simulink model "Noa_Nofusion_backup"  (R2020b)
settings: Solver=FixedStepDiscrete  StartTime=0.0  StopTime=Inf  FixedStep=0.02  RelTol=1e-3
PostLoadFcn:
  | if any(exist('dsrtsu_mdlpostloadfcn', 'file') ~= 0), dsrtsu_mdlpostloadfcn('Execute', bdroot); end
InitFcn:
  | , if any(exist('rtifpga_mdlclblib', 'file') ~= 0), rtifpga_mdlclblib('Init', bdroot); end,
  | , if any(exist('dsmpb_private', 'file') ~= 0), dsmpb_private('dsmpb_mdlclblib', 'Init', bdroot); end,
undefined symbols (not defined in the file): ACC_TimeGap_DecSetSwt, ACC_TimeGap_IncSetSwt, AccelPedalPosn, AccelPedalPosnVldty, AccelPedlPosnDiagc, AccPedalOverride, ACU_ShiftInProgress, ADAS_Posn_CurLane, AESSwtReq, ALC_SwtReq, BrkPedalSts, CC_ACC_CANCEL_OFFSwt, CC_ACC_CRUISE_OFFSwt, CC_ACC_DecSetSpd_SetSwt, CC_ACC_IncSetSpd_ResuSwt, CC_ACCSwtErr, CharSpd_ms, CSA_NODE, CURRENT_GEAR, CurrentGearValid, DiscIntNeverNeededParam, DrvDoorSts, DrvSBR, DrvTrqReqOvld, ECMACCInterface, ECMRespACC, ELKSwtReq, EngLimpHomeSts, EngSpd, EngState, EngState_PHEV, EngTrqMaxActSpd, EngTrqMinAct, EPS_DrvInpTrqVal_HighReslolution, EPS_FailSts, EPS_LKATorqOvrlDlvd, EPS_LKATorqOvrlDlvdVld, EPS_LKATrqOvlDlvdSts, EPS_SteerMod, EPS_TrqSnsrSts, EQ4_APPINFO, EQ4_LA_ELEM, EQ4_LA_HDR, EQ4_LAP_ELEM, EQ4_LAP_HDR, EQ4_LH_ELEM, EQ4_LH_HDR, EQ4_LRE_ELEM, EQ4_LRE_HDR, ESS_PedSwtReq, ESS_VehSwtReq, FFogLmpSts_F_Pbox, FLWheelDriveDirection, FLWheelSpd, FrntWiprSwtSts, FrntWshrSwtSts, FRWheelDriveDirection, FRWheelSpd, HazardLmpSwtSts, HCU_AccelPedalPosn_Diag ... (+152)
libraries: simulink x117, dsmpblib x30
(part 10 of 11)

== matlab function Noa_Nofusion_backup/Subsystem2/ACCOSM/HWA_Task100ms1/Trajectory/Trajectory/CalcEgoVehMove ==
  data: dDeltaX output single size=1; tCycle input size=1; Kap input size=1; Vego input size=1; alpSideSlipAngle input size=1; dDeltaY output single size=1; CosOfPsi output single size=1; SinOfPsi output single size=1; WheelTrack input; SlipDislim output; Vch input
function [dDeltaX,dDeltaY,CosOfPsi,SinOfPsi,SlipDislim] = EgoVehicleMovement(tCycle,Kap,Vego,alpSideSlipAngle,WheelTrack,Vch)
%#codegen
if Kap==0
    dDeltaX = Vego*tCycle;
    dDeltaY = single(0);
    CosOfPsi = single(1);
    SinOfPsi = single(0);
    SlipDislim = Vch*1000;
else
    SlipDislim = max(WheelTrack*1000,min(tCycle*Vego,Kap*15));
    t_Psi = Kap*Vego*tCycle;
    SinOfPsi = sin(t_Psi);
    CosOfPsi = cos(t_Psi);
    t_dDeltaXTemp = SinOfPsi/Kap;
    t_dDeltaYTemp = 2*(sin(t_Psi/2)*sin(t_Psi/2))/Kap;
    dDeltaX = min(cos(alpSideSlipAngle)*t_dDeltaXTemp - sin(alpSideSlipAngle)*t_dDeltaYTemp,SlipDislim);
    dDeltaY = sin(alpSideSlipAngle)*t_dDeltaXTemp + cos(alpSideSlipAngle)*t_dDeltaYTemp;
end

== matlab function Noa_Nofusion_backup/Subsystem2/ACCOSM/HWA_Task100ms1/Trajectory/Trajectory/Priority ==
  data: ObjNumber input; ObjValid input; ObjPrio output single; ObjClass input; ObjDx input; ObjMatrix output single
function [ObjPrio,ObjMatrix] = fcn(ObjNumber,ObjValid,ObjClass,ObjDx)
%#codegen
ObjPrio = single(zeros(15,1));

for i=1:ObjNumber
    if ObjValid(i)
        if ObjDx(i)<0
            ObjPrio(i)=single(0);
        else
            if (ObjClass(i)==2)||(ObjClass(i)==3)||(ObjClass(i)==5)
                t_ObjPrio=single(2*255);
            else
                t_ObjPrio=single(255);
            end
            ObjPrio(i) = t_ObjPrio - ObjDx(i);
        end
    else
        ObjPrio(i)=single(0);
    end
end

ObjMatrix=ObjPrio;

t_h=1;
while 1
    t_h = t_h*3+1;
    if t_h>=ObjNumber
        break;
    end
end

%   t_h = 121;
while 1
    t_h = fix(t_h/3);
    for i=(t_h+1):ObjNumber
        j=i;
        t_zw=ObjMatrix(i);
        while (j>t_h)&&(t_zw<ObjMatrix(j-t_h))
            ObjMatrix(j)=ObjMatrix(j-t_h);
            j=j-t_h;
        end
        ObjMatrix(j)=t_zw;
    end
    if t_h==1
        break;
    end
end

== matlab function Noa_Nofusion_backup/Subsystem2/ACCOSM/HWA_Task100ms1/Trajectory/Trajectory/ReleaseLowPriorityObjects ==
  data: TrajUsed output; ObjNumber input; TrajNumber input; ObjPrio input; ObjMatrix input; ObjValid input; TrajCurrentIndex input; TrajUsedK1 input; TrajHistBufferBTrajEndK1 input; ObjTrajNumberK1 input; TrajHistBufferBTrajEnd output; ObjTrajNumber output
function [TrajUsed,TrajHistBufferBTrajEnd,ObjTrajNumber] =...
    fcn(ObjNumber,TrajNumber,ObjPrio,ObjMatrix,ObjValid,TrajCurrentIndex,...
    TrajUsedK1,TrajHistBufferBTrajEndK1,ObjTrajNumberK1)
%#codegen
TrajHistBufferBTrajEnd = TrajHistBufferBTrajEndK1;
TrajUsed = TrajUsedK1;
ObjTrajNumber = ObjTrajNumberK1;
ObjPrioLimit = ObjMatrix(ObjNumber-TrajNumber);

for i=1:ObjNumber
    if ObjValid(i)
        if (ObjPrio(i)==0)||(ObjPrio(i)<=ObjPrioLimit)
            j = ObjTrajNumber(i);
            if j<(TrajNumber+1)
                t = TrajCurrentIndex(j);
                TrajHistBufferBTrajEnd(j,t)=1;
                TrajUsed(j)=0;
                ObjTrajNumber(i)=255;
            end
        end
    end
end

== matlab function Noa_Nofusion_backup/Subsystem2/ACCOSM/HWA_Task100ms1/Trajectory/Trajectory/StoreEgoTrajectory ==
  data: Pa output single; Pb output single; Pc output single; Pd output single; BufNumber input; tCycle input; EgoTrajHistCurrentIndex output uint8; EgoDDeltaX input; EgoDDeltaY input; EgoCosOfPsi input; EgoSinOfPsi input; EgoTrajHistDxv output; EgoTrajHistDyv output; EgoTrajHistTTimeStamp output; EgoTrajHistCurrentIndexK1 input; EgoTrajHistDxvK1 input single; EgoTrajHistDyvK1 input single; EgoTrajHistTTimeStampK1 input single
function [Pa,Pb,Pc,Pd,EgoTrajHistCurrentIndex,EgoTrajHistDxv,EgoTrajHistDyv,EgoTrajHistTTimeStamp]...
    = fcn(BufNumber,tCycle,EgoDDeltaX,EgoDDeltaY,EgoCosOfPsi,EgoSinOfPsi,...
    EgoTrajHistCurrentIndexK1,EgoTrajHistDxvK1,EgoTrajHistDyvK1,EgoTrajHistTTimeStampK1)
%#codegen
EgoTrajHistCurrentIndex = EgoTrajHistCurrentIndexK1;
EgoTrajHistDxv = EgoTrajHistDxvK1;
EgoTrajHistDyv = EgoTrajHistDyvK1;
EgoTrajHistTTimeStamp = EgoTrajHistTTimeStampK1;
% alpWheelAngleOffset = alpWheelAngleOffsetK1;

t_IdxActualElement = EgoTrajHistCurrentIndex;
if t_IdxActualElement==BufNumber
    t_IdxNextElement=uint8(1);
else
    t_IdxNextElement=t_IdxActualElement+1;
end

Temp1 = EgoTrajHistDxv(t_IdxActualElement) - EgoDDeltaX;
Temp2 = EgoTrajHistDyv(t_IdxActualElement) - EgoDDeltaY;
dDeltaS = Temp1*Temp1 + Temp2*Temp2;
t_AddPosition = ((EgoTrajHistTTimeStamp(t_IdxActualElement)+tCycle)>0.3);
t_AddPosition = t_AddPosition&(dDeltaS>4);
t_AddPosition = t_AddPosition|(dDeltaS>100);
for iBuf=1:BufNumber
    if (t_AddPosition==1)&&(iBuf==t_IdxNextElement)
        EgoTrajHistDxv(iBuf)=single(0);
        EgoTrajHistDyv(iBuf)=single(0);
        EgoTrajHistTTimeStamp(iBuf)=single(0);
        EgoTrajHistCurrentIndex = t_IdxNextElement;
    else
        dX = EgoTrajHistDxv(iBuf)-EgoDDeltaX;
        dY = EgoTrajHistDyv(iBuf)-EgoDDeltaY;
        if (EgoTrajHistDxv(iBuf)>-255)&&(dX>-255)&&(dX<255)&&(dY>-255)&&(dY<255)
            Temp1 = dX*EgoCosOfPsi + dY*EgoSinOfPsi;
            Temp2 = -dX*EgoSinOfPsi + dY*EgoCosOfPsi;
            if (Temp1>-255)&&(Temp1<255)&&(Temp2>-255)&&(Temp2<255)
                EgoTrajHistDxv(iBuf)=Temp1;
                EgoTrajHistDyv(iBuf)=Temp2;
                tDt = EgoTrajHistTTimeStamp(iBuf)+tCycle;
                if tDt>32
                    tDt=single(32);
                end
                EgoTrajHistTTimeStamp(iBuf) = tDt;
            else
                EgoTrajHistDxv(iBuf)=single(-255);
                EgoTrajHistDyv(iBuf)=single(-255);
                EgoTrajHistTTimeStamp(iBuf) = single(32);
            end
        else
            EgoTrajHistDxv(iBuf)=single(-255);
            EgoTrajHistDyv(iBuf)=single(-255);
            EgoTrajHistTTimeStamp(iBuf) = single(32);
        end
    end
end

t_Index = EgoTrajHistCurrentIndex;
t_Index1 = BufNumber + uint8(23);
t_Index2 = BufNumber + uint8(21);
t_Index3 = BufNumber + uint8(19);

if t_Index1>24
    t_Index1 = t_Index1 - uint8(24);
end
if t_Index2>24
    t_Index2 = t_Index2 - uint8(24);
end
if t_Index3>24
    t_Index3 = t_Index3 - uint8(24);
end

XiMa = [EgoTrajHistDxv(t_Index);EgoTrajHistDxv(t_Index1);EgoTrajHistDxv(t_Index2);EgoTrajHistDxv(t_Index3)];
YiMa = [EgoTrajHistDyv(t_Index);EgoTrajHistDyv(t_Index1);EgoTrajHistDyv(t_Index2);EgoTrajHistDyv(t_Index3)];

[Pa,Pb,Pc,Pd] = pl(XiMa,YiMa);

% if (abs(EgoTrajHistDyv(t_Index1))<0.1)&&(abs(EgoTrajHistDyv(t_Index2))<0.1)&&(abs(EgoTrajHistDyv(t_Index3))<0.1)
%     kapRef = 3*Pa*EgoTrajHistDxv(t_Index2) + 2*Pb;
%     AckConst = min((1+VxvRef*VxvRef/(26*26))*2.68/max(VxvRef,1),32767);
%     alpWheelAngleRef = VxvRef*kapRef*AckConst;
%     Raw = alpWheelAngleMean - alpWheelAngleRef;
%     if VxvRef>7.3
%         alpWheelAngleOffset = (Raw - alpWheelAngleOffset)/10000 + alpWheelAngleOffset;
%     end
% else
%     alpWheelAngleRef = single(255);
% end

== matlab function Noa_Nofusion_backup/Subsystem2/ACCOSM/HWA_Task100ms1/VycCalc ==
  data: ObjVyc output single size=15; dxC0 input; aP0 input; bP0 input; aP1 input; bP1 input; ObjValid input boolean size=15; ObjDx input single size=15; ObjVxG input single size=15; ObjVyG input single size=15; ObjYawAngle output
function [ObjVyc,ObjYawAngle] = VycCalc(dxC0,aP0,bP0,aP1,bP1,ObjValid,ObjDx,ObjVxG,ObjVyG)

ObjVyc = single(zeros(15,1));
ObjYawAngle = single(zeros(15,1));

for i=1:15
    if ObjValid(i)
       t_dxv = ObjDx(i);
       t_VxG = ObjVxG(i);
       t_VyG = ObjVyG(i);
       
       if abs(t_VxG)<0.1
          if t_VyG>0.5
              ObjYawAngle(i) = single(1.57);
          end
          if t_VyG<-0.5
              ObjYawAngle(i) = single(-1.57);
          end
       else
           if t_VxG>0
               ObjYawAngle(i) = atan(t_VyG/t_VxG);
           else
               if t_VyG>0
                  ObjYawAngle(i) = single(3.1416) + atan(t_VyG/t_VxG);
               else
                  ObjYawAngle(i) = -single(3.1416) + atan(t_VyG/t_VxG);
               end
           end
       end
       
       t_bParabolaYNLane = single(1);
       if t_dxv<dxC0
          temp1 =  2*aP0*t_dxv + bP0;
          t_bParabolaXNLane = -temp1;
       else
          temp1 =  2*aP1*t_dxv + bP1;
          t_bParabolaXNLane = -temp1;
       end
       t_bParabolaMag = mag(t_bParabolaXNLane,t_bParabolaYNLane);
       t_bParabolaXNLane = t_bParabolaXNLane/t_bParabolaMag;
       t_bParabolaYNLane = t_bParabolaYNLane/t_bParabolaMag;
       temp1 = t_VxG*t_bParabolaXNLane;
       temp2 = t_VyG*t_bParabolaYNLane;
       
       ObjVyc(i) = temp1 + temp2;
    else
       ObjVyc(i) = single(0);
    end
end
end

function out = mag(x,y)
M = max(abs(x),abs(y));
N = min(abs(x),abs(y));
out = M + 0.322*N;
end

== matlab function Noa_Nofusion_backup/Subsystem2/ACCOSM/HWA_Task100ms1/dyLaneWidthSteerAdapt ==
  data: kap input; dyLaneAdaptLeft output; dyAdapt input; dyLaneAdaptRight output
function [dyLaneAdaptLeft,dyLaneAdaptRight] = fcn(kap,dyAdapt)

dyLaneAdaptLeft = single(0);
dyLaneAdaptRight = single(0);
if kap>0
    dyLaneAdaptRight = dyAdapt;
end
if kap<0
    dyLaneAdaptLeft = dyAdapt;
end

== matlab function Noa_Nofusion_backup/Subsystem2/ACCOSM/HWA_Task100ms1/wCutInVy ==
  data: DycASI output single; ObjValid input boolean size=15; ObjDycCutIn input single size=15; ObjWidth input single size=15; ObjVyc input single size=15; ObjDx input single size=15; ObjDy input single size=15; ObjCnt input uint8 size=15; ObjDycFilt input single size=15; ObjwCutInVyK1 input single size=15; ObjtPrediction4CutIn output single size=15; ObjDycCutInPredict output single size=15; ObjCutIn_b output boolean size=15; ObjwCutInVy output single size=15
function [DycASI,ObjtPrediction4CutIn,ObjDycCutInPredict,ObjCutIn_b,ObjwCutInVy] = ...
    CalcWCutInVy(ObjValid,ObjDycCutIn,ObjWidth,ObjVyc,ObjDx,ObjDy,ObjCnt,...
    ObjDycFilt,ObjwCutInVyK1)
 
ObjwCutInVy = single(zeros(15,1));
ObjtPrediction4CutIn = single(zeros(15,1));
ObjDycCutInPredict = single(zeros(15,1));
DycASI = single(zeros(15,1));
ObjCutIn_b = false(15,1);
 
for i=1:15
    if ObjValid(i)
        dWidth = ObjWidth(i);
        dycASI = ObjDycCutIn(i);
        vyc = ObjVyc(i);
        dx = ObjDx(i);
        dy = ObjDy(i);
        dycFilt = ObjDycFilt(i);
        wCutInVyK1 = ObjwCutInVyK1(i);
  
        temp1 = dycFilt - dycASI;
        if ((dycASI>0)&&(temp1>0.2))||((dycASI<0)&&(temp1<-0.2))
            tauVy = single(1.6);
        else
            tauVy = single(0);
        end
        tauVy = interpolate(single(40),tauVy,single(70),single(0),dx);
        ObjtPrediction4CutIn(i) = tauVy;
        temp1 = vyc*tauVy;
        temp2 = dycASI + temp1;
        
        if (dycASI>0)&&(temp2<0)
            temp2 = single(0);
        else
            if (dycASI<0)&&(temp2>0)
                temp2 = single(0);
            else
                if dycASI==0
                    temp2 = single(0);
                end
            end
        end
        ObjDycCutInPredict(i) = temp2;
        if dycASI>0
            temp1 = temp2 - 0.5*dWidth;
            t_dycASI = max(temp1,single(0));
        else
            temp1 = temp2 + 0.5*dWidth;
            t_dycASI = min(temp1,single(0));
        end
        temp1 = abs(t_dycASI);
        t_wCutInVy = interpolate(single(0),single(1),single(0.7),single(0),temp1);
        if tauVy==0
            t_wCutInVy = single(0);
        end
        
        if dx>0
            fak = abs(dy)/dx; 
        else
            fak = single(0);
        end
        if (ObjCnt(i)<2)||(abs(dy)>=2.4)||(fak>0.25)
           t_wCutInVy = single(0);
        end
       
        temp1 = t_wCutInVy - wCutInVyK1;
        temp1_ub = abs(temp1);
        temp2 = 0.2*temp1_ub;
        if temp1>0
            t_wCutInVy = wCutInVyK1 + temp2;
        else
            t_wCutInVy = wCutInVyK1 - temp2;
        end
        ObjwCutInVy(i) = t_wCutInVy;
        DycASI(i) = t_dycASI;
        if t_wCutInVy>0.7
            ObjCutIn_b(i) = true;
        end
    end
end
end
 
% function out = interpolate(x1,z1,x2,z2,Raw)
% if Raw<=x1
%     out = z1;
% else
%     if Raw>=x2
%         out = z2;
%     else
%         out = z1 + (Raw-x1)*(z2-z1)/(x2-x1);
%     end
% end
% end

== matlab function Noa_Nofusion_backup/Subsystem2/ACCOSM/HWA_Task100ms1/wCutOutVy ==
  data: vRef input single size=1; kap input single size=1; tDirIndLeft input single size=1; tDirIndRight input single size=1; ObjValid input boolean size=15; ObjDycCutIn input single size=15; ObjWidth input single size=15; ObjtPrediction4CutOut output single size=15; ObjDycCutOutPredict output single size=15; ObjwCutOutTurnOff output single size=15; ObjVyc input single size=15; ObjDx input single size=15; ObjDy input single size=15; ObjVx input single size=15; ObjVy input single size=15; ObjDyc input single size=15; ObjDrive_b input boolean size=15; ObjCnt input uint8 size=15; ObjDycFilt input single size=15; ObjwCutoutVyK1 input single size=15; ObjwCutoutVy output single size=15
function [ObjtPrediction4CutOut,ObjDycCutOutPredict,ObjwCutOutTurnOff,ObjwCutoutVy] = ...
    CalcWCutOutVy(vRef,kap,tDirIndLeft,tDirIndRight,ObjValid,ObjDycCutIn,ObjWidth,...
    ObjVyc,ObjDx,ObjDy,ObjVx,ObjVy,ObjDyc,ObjDrive_b,ObjCnt,...
    ObjDycFilt,ObjwCutoutVyK1)
 
ObjwCutoutVy = single(zeros(15,1));
ObjtPrediction4CutOut = single(zeros(15,1));
ObjDycCutOutPredict = single(zeros(15,1));
ObjwCutOutTurnOff = single(zeros(15,1));
 
for i=1:15
    if ObjValid(i)
        dWidth = ObjWidth(i);
        dycASI = ObjDycCutIn(i);
        vyc = ObjVyc(i);
        dx = ObjDx(i);
        dy = ObjDy(i);
        vx = ObjVx(i);
        vy = ObjVy(i);
        dyc = ObjDyc(i);
        dycFilt = ObjDycFilt(i);
        wCutoutVyK1 = ObjwCutoutVyK1(i);
        Move_b = ObjDrive_b(i);
        Cnt = ObjCnt(i);
        t_vxTO = vRef + vx;
        t_vxvThreshold = 0.5 - vRef;
        
        temp1 = dycASI - dycFilt;
        if ((dycASI>0)&&(temp1>0.2))||((dycASI<0)&&(temp1<-0.2))
            tauVy = single(1);
        else
            tauVy = single(0);
        end
        tauVy = interpolate(single(40),tauVy,single(70),single(0),dx);
        ObjtPrediction4CutOut(i) = tauVy;
        temp1 = vyc*tauVy;
        temp2 = dycASI + temp1;
        
        if (dycASI>0)&&(temp2<0)
            temp2 = single(0);
        else
            if (dycASI<0)&&(temp2>0)
                temp2 = single(0);
            else
                if dycASI==0
                    temp2 = single(0);
                end
            end
        end
        ObjDycCutOutPredict(i) = temp2;
        if dycASI>0
            temp1 = temp2 + 0.5*dWidth;
            t_dycASI = max(temp1,single(0));
        else
            temp1 = temp2 - 0.5*dWidth;
            t_dycASI = min(temp1,single(0));
        end
        temp1 = abs(t_dycASI);
        t_wCutoutVy = interpolate(single(0),single(0),single(0.7),single(1),temp1);
        if tauVy==0
            t_wCutoutVy = single(0);
        end
        
        temp1 = t_wCutoutVy - wCutoutVyK1;
        temp1_ub = abs(temp1);
        temp2 = 0.2*temp1_ub;
        if temp1>0
            t_wCutoutVy = wCutoutVyK1 + temp2;
        else
            t_wCutoutVy = wCutoutVyK1 - temp2;
        end
        ObjwCutoutVy(i) = t_wCutoutVy;
        if (dx<30)&&(Move_b==true)&&(vRef>0.5)&&(t_vxTO<6)&&(vx>t_vxvThreshold)&&(abs(dyc)>0.5)&&...
        (abs(dy)>0.5)&&(abs(dy)<4)&&(abs(vy)>0.5)&&...
        (((dyc<0)&&(vyc<0)&&(tDirIndRight==0))||((dyc>0)&&(vyc>0)&&(tDirIndLeft==0)))&&...
        (kap>-0.005)&&(kap<0.005)&&...
        (Cnt==7) 
             ObjwCutOutTurnOff(i) = t_wCutoutVy;
        end
    end
end
end

== matlab function Noa_Nofusion_backup/CR_RSDS_Input/CL ==
  data: ID input uint8 size=11; Dx input single size=11; Dy input single size=11; Vx input single size=11; Vy input single size=11; Ax input single size=11; Age input uint8 size=11; MoveSts input uint8 size=11; FusType input uint8 size=11; ObjIDK1 input uint8 size=11; ObjDx output single size=11; ObjDy output single size=11; ObjVx output single size=11; ObjVy output single size=11; ObjAx output single size=11; ObjAge output uint8 size=11; ObjMoveSts output uint8 size=11; ObjFusType output uint8 size=11; ObjID output uint8 size=11
function [ObjDx,ObjDy,ObjVx,ObjVy,ObjAx,ObjAge,ObjMoveSts,ObjFusType,ObjID] =...
    DataT(ID,Dx,Dy,Vx,Vy,Ax,Age,MoveSts,FusType,ObjIDK1)

ObjID = uint8(zeros(11,1));
ObjDx = single(zeros(11,1));
ObjDy = single(zeros(11,1));
ObjVx = single(zeros(11,1));
ObjVy = single(zeros(11,1));
ObjAx = single(zeros(11,1));
ObjAge = uint8(zeros(11,1));
ObjMoveSts = uint8(zeros(11,1));
ObjFusType = uint8(zeros(11,1));

T = uint8(zeros(11,1));
P = uint8(zeros(11,1));
Index01 = uint8(zeros(11,1));
Index02 = uint8(zeros(11,1));
M = uint8(0);
N = uint8(0);
w = uint8(0);

for i=uint8(1):uint8(11)
    for j=uint8(1):uint8(11)
        if ID(i)==ObjIDK1(j) && ID(i)>uint8(0)
            T(j) = i;
            P(i) = j;
        end
    end
end

for j=uint8(1):uint8(11)
    if T(j)==uint8(0)
        if ObjIDK1(j)==uint8(0)
            N = N + uint8(1);
            Index01(N) = j;
        else
            M = M + uint8(1);
            Index02(M) = j;
        end
    end
end

for i=uint8(1):uint8(11)
    if P(i)==uint8(0) && ID(i)>uint8(0)
        w = w + uint8(1);
        if w<=N
            P(i) = Index01(w);
        else
            P(i) = Index02(w - N);
        end
    end
    if P(i)>uint8(0)
       ObjID(P(i)) = ID(i);
       ObjDx(P(i)) = Dx(i);
       ObjDy(P(i)) = Dy(i);
       ObjVx(P(i)) = Vx(i);
       ObjVy(P(i)) = Vy(i);
       ObjAx(P(i)) = Ax(i);
       ObjAge(P(i)) = Age(i);
       ObjMoveSts(P(i)) = MoveSts(i);
       ObjFusType(P(i)) = FusType(i);
    end
end
end

== matlab function Noa_Nofusion_backup/CR_RSDS_Input/CR_L_Bus/CL ==
  data: RadarID input uint8 size=1; ID input uint8 size=6; Dx input single size=6; Dy input single size=6; Vx input single size=6; Vy input single size=6; Ax input single size=6; ObjIDK1 input uint8 size=6; P output uint8 size=6; ObjDx output single size=6; ObjDy output single size=6; ObjVx output single size=6; ObjVy output single size=6; ObjAx output single size=6; ObjMoveSts output uint8 size=6; ObjFusType output uint8 size=6; ObjID output uint8 size=6; ObjAgeK1 input uint8 size=6; ObjAge output uint8 size=6
function [P,ObjDx,ObjDy,ObjVx,ObjVy,ObjAx,ObjMoveSts,ObjFusType,ObjID,ObjAge] =...
    DataT(RadarID,ID,Dx,Dy,Vx,Vy,Ax,ObjIDK1,ObjAgeK1)

if RadarID==uint8(1)
    FusFac = 4;
elseif RadarID==uint8(2)
    FusFac = 8;
elseif RadarID==uint8(3)
    FusFac = 16;
else
    FusFac = 32;
end

ObjID = uint8(zeros(6,1));
ObjDx = single(zeros(6,1));
ObjDy = single(zeros(6,1));
ObjVx = single(zeros(6,1));
ObjVy = single(zeros(6,1));
ObjAx = single(zeros(6,1));
ObjAge = uint8(ones(6,1));
ObjMoveSts = uint8(2*ones(6,1));
ObjFusType = uint8(FusFac*ones(6,1));

T = uint8(zeros(6,1));
P = uint8(zeros(6,1));
Index01 = uint8(zeros(6,1));
Index02 = uint8(zeros(6,1));
M = uint8(0);
N = uint8(0);
w = uint8(0);

for i=uint8(1):uint8(6)
    for j=uint8(1):uint8(6)
        if ID(i)==ObjIDK1(j) && ID(i)>uint8(0)
            T(j) = i;
            P(i) = j;
        end
    end
end

for j=uint8(1):uint8(6)
    if T(j)==uint8(0)
        if ObjIDK1(j)==uint8(0)
            N = N + uint8(1);
            Index01(N) = j;
        else
            M = M + uint8(1);
            Index02(M) = j;
        end
    end
end

for i=uint8(1):uint8(6)
    if P(i)==uint8(0) && ID(i)>uint8(0)
        w = w + uint8(1);
        if w<=N
            P(i) = Index01(w);
        else
            P(i) = Index02(w - N);
        end
    elseif P(i)>uint8(0)
        ObjAge(P(i)) = min(ObjAgeK1(i) + uint8(1),uint8(255));
    end
    if P(i)>uint8(0)
       ObjID(P(i)) = ID(i);
       ObjDx(P(i)) = Dx(i);
       ObjDy(P(i)) = Dy(i);
       ObjVx(P(i)) = Vx(i);
       ObjVy(P(i)) = Vy(i);
       ObjAx(P(i)) = Ax(i);
    end
end
for i=uint8(1):uint8(6)
    if ObjID(i)==uint8(0)
        ObjAge(i) = uint8(0);
        ObjMoveSts(i) = uint8(0);
        ObjFusType(i) = uint8(0);
    end
end
end

== matlab function Noa_Nofusion_backup/CR_RSDS_Input/CR_R_Bus/CR ==
  data: RadarID input uint8 size=1; ID input uint8 size=6; Dx input single size=6; Dy input single size=6; Vx input single size=6; Vy input single size=6; Ax input single size=6; ObjIDK1 input uint8 size=6; P output uint8 size=6; ObjDx output single size=6; ObjDy output single size=6; ObjVx output single size=6; ObjVy output single size=6; ObjAx output single size=6; ObjMoveSts output uint8 size=6; ObjFusType output uint8 size=6; ObjID output uint8 size=6; ObjAgeK1 input uint8 size=6; ObjAge output uint8 size=6
function [P,ObjDx,ObjDy,ObjVx,ObjVy,ObjAx,ObjMoveSts,ObjFusType,ObjID,ObjAge] =...
    DataT(RadarID,ID,Dx,Dy,Vx,Vy,Ax,ObjIDK1,ObjAgeK1)

if RadarID==uint8(1)
    FusFac = 4;
elseif RadarID==uint8(2)
    FusFac = 8;
elseif RadarID==uint8(3)
    FusFac = 16;
else
    FusFac = 32;
end

ObjID = uint8(zeros(6,1));
ObjDx = single(zeros(6,1));
ObjDy = single(zeros(6,1));
ObjVx = single(zeros(6,1));
ObjVy = single(zeros(6,1));
ObjAx = single(zeros(6,1));
ObjAge = uint8(ones(6,1));
ObjMoveSts = uint8(2*ones(6,1));
ObjFusType = uint8(FusFac*ones(6,1));

T = uint8(zeros(6,1));
P = uint8(zeros(6,1));
Index01 = uint8(zeros(6,1));
Index02 = uint8(zeros(6,1));
M = uint8(0);
N = uint8(0);
w = uint8(0);

for i=uint8(1):uint8(6)
    for j=uint8(1):uint8(6)
        if ID(i)==ObjIDK1(j) && ID(i)>uint8(0)
            T(j) = i;
            P(i) = j;
        end
    end
end

for j=uint8(1):uint8(6)
    if T(j)==uint8(0)
        if ObjIDK1(j)==uint8(0)
            N = N + uint8(1);
            Index01(N) = j;
        else
            M = M + uint8(1);
            Index02(M) = j;
        end
    end
end

for i=uint8(1):uint8(6)
    if P(i)==uint8(0) && ID(i)>uint8(0)
        w = w + uint8(1);
        if w<=N
            P(i) = Index01(w);
        else
            P(i) = Index02(w - N);
        end
    elseif P(i)>uint8(0)
        ObjAge(P(i)) = min(ObjAgeK1(i) + uint8(1),uint8(255));
    end
    if P(i)>uint8(0)
       ObjID(P(i)) = ID(i);
       ObjDx(P(i)) = Dx(i);
       ObjDy(P(i)) = Dy(i);
       ObjVx(P(i)) = Vx(i);
       ObjVy(P(i)) = Vy(i);
       ObjAx(P(i)) = Ax(i);
    end
end
for i=uint8(1):uint8(6)
    if ObjID(i)==uint8(0)
        ObjAge(i) = uint8(0);
        ObjMoveSts(i) = uint8(0);
        ObjFusType(i) = uint8(0);
    end
end
end

== matlab function Noa_Nofusion_backup/Subsystem2/ACCOSM/ObjMatrixTransit/Subsystem/MATLAB Function1 ==
  data: P output uint8; Count input uint8 size=1; ID input uint8 size=20; BrakeLight_b input uint8 size=20; Class input uint8 size=20; LatDis input single size=20; LatVel input single size=20; LongAccel input single size=20; LongDis input single size=20; LongVel input single size=20; Width input single size=20; Age input uint16 size=20; MotionSts input uint8 size=20; ObjValid output boolean size=20; ObjBrakeLightIndic output uint8 size=20; ObjClassification output uint8 size=20; ObjLatPos output single size=20; ObjLatVel output single size=20; ObjLongAccel output single size=20; ObjLongVel output single size=20; ObjWidth output single size=20; ObjCnt output uint8 size=20; ObjMoveSts output uint8 size=20; ObjLongPos output single size=20; ObjIDK1 input uint8 size=20; ObjID output uint8 size=20
function [P,ObjValid,ObjBrakeLightIndic,ObjClassification,...
    ObjLatPos,ObjLatVel,ObjLongAccel,ObjLongVel,...
    ObjWidth,ObjCnt,ObjMoveSts,ObjLongPos,ObjID] =...
    DataT(Count,ID,BrakeLight_b,Class,LatDis,LatVel,LongAccel,LongDis,LongVel,Width,Age,MotionSts,ObjIDK1)

ObjValid = false(20,1);
ObjID = uint8(zeros(20,1));
ObjBrakeLightIndic = uint8(zeros(20,1));
ObjClassification = uint8(zeros(20,1));
ObjLatPos = single(zeros(20,1));
ObjLatVel = single(zeros(20,1));
ObjLongAccel = single(zeros(20,1));
ObjLongPos = single(zeros(20,1));
ObjLongVel = single(zeros(20,1));
ObjWidth = single(zeros(20,1));
ObjCnt = uint8(zeros(20,1));
ObjMoveSts = uint8(zeros(20,1));

T = uint8(zeros(20,1));
P = uint8(zeros(20,1));
Index01 = uint8(zeros(20,1));
Index02 = uint8(zeros(20,1));
M = uint8(0);
N = uint8(0);
w = uint8(0);

for i=uint8(1):Count
    for j=uint8(1):uint8(20)
        if ID(i)==ObjIDK1(j)
            T(j) = i;
            P(i) = j;
        end
    end
end

for j=uint8(1):uint8(20)
    if T(j)==uint8(0)
        if ObjIDK1(j)==uint8(0)
            N = N + uint8(1);
            Index01(N) = j;
        else
            M = M + uint8(1);
            Index02(M) = j;
        end
        ObjValid(j) = false;
    else
        ObjValid(j) = true;
    end
end

for i=uint8(1):Count
    if P(i)==uint8(0)
        w = w + uint8(1);
        if w<=N
            P(i) = Index01(w);
        else
            P(i) = Index02(w - N);
        end
        ObjValid(Index01(w)) = true;
    end
    ObjID(P(i)) = ID(i);
    if BrakeLight_b(i)==uint8(1)
        ObjBrakeLightIndic(P(i)) = uint8(2);
    end
    if Class(i)==uint8(1)||Class(i)==uint8(2)||...
            Class(i)==uint8(3)||Class(i)==uint8(6)
        ObjClassification(P(i)) = uint8(1);
    end
    ObjLatPos(P(i)) = -LatDis(i) - single(0.1);
    ObjLatVel(P(i)) = -LatVel(i);
    ObjLongAccel(P(i)) = LongAccel(i);
    ObjLongPos(P(i)) = LongDis(i);
    ObjLongVel(P(i)) = LongVel(i);
    ObjWidth(P(i)) = Width(i);
    if Age(i)<=255
        ObjCnt(P(i)) = uint8(Age(i)/2) - uint8(1);
    else
        ObjCnt(P(i)) = uint8(127);
    end
    if MotionSts(i)==uint8(1)||MotionSts(i)==uint8(3)
        ObjMoveSts(P(i)) = uint8(1);
    elseif MotionSts(i)==uint8(2)||MotionSts(i)==uint8(5)
        if LongVel(i)>-2.5
            ObjMoveSts(P(i)) = uint8(2);
        else
            ObjMoveSts(P(i)) = uint8(4);
        end
    elseif MotionSts(i)==uint8(4)
        ObjMoveSts(P(i)) = uint8(3);
    end
end
end

== stateflow chart Noa_Nofusion_backup/Subsystem2/ACCOSM/ObjMatrixTransit/Subsystem/Obj ==
  (default) -> (junction 5)
  (junction 5) -> (junction 36) : {i=1;}
  (junction 36) -> (junction 38) [order 1] : [i<21]
  (junction 40) -> (junction 36) : {i=i+1;}
  (junction 36) -> (junction 42) [order 2]
  (junction 38) -> (junction 40) : {id(i) = IFV410_Obj(i).OBJ_ID;
      | confidence(i) = IFV410_Obj(i).OBJ_Existence_Probability;
      | classification(i) = IFV410_Obj(i).OBJ_Object_Class;
      | width(i) = IFV410_Obj(i).OBJ_Width;
      | LongDis(i) = IFV410_Obj(i).OBJ_Long_Distance;
      | LatDis(i) = IFV410_Obj(i).OBJ_Lat_Distance;
      | AbsLongAcc(i) = IFV410_Obj(i).OBJ_Abs_Long_Acc;
      | AbsLongVel(i) = IFV410_Obj(i).OBJ_Abs_Long_Velocity;
      | AbsLatVel(i) = IFV410_Obj(i).OBJ_Abs_Lat_Velocity;
      | BrakeLight(i) = IFV410_Obj(i).OBJ_Brake_Light;
      | Age(i) = IFV410_Obj(i).OBJ_Object_Age;
      | motionSts(i) = IFV410_Obj(i).OBJ_Motion_Status;
      | motionCategory(i) = IFV410_Obj(i).OBJ_Motion_Category;
      | motionOrientation(i) = IFV410_Obj(i).OBJ_Motion_Orientation;}
  data: i local uint8; id output uint8 size=20 =uint8(zeros(20,1)); classification output uint8 size=20 =uint8(zeros(20,1)); AbsLongAcc output single size=20 =single(zeros(20,1)); width output single size=20 =single(zeros(20,1)); AbsLongVel output single size=20 =single(zeros(20,1)); LongDis output single size=20 =single(zeros(20,1)); AbsLatVel output single size=20 =single(zeros(20,1)); LatDis output single size=20 =single(zeros(20,1)); BrakeLight output uint8 size=20 =uint8(zeros(20,1)); Age output uint16 size=20 =uint16(zeros(20,1)); confidence output single size=20 =single(zeros(20,1)); IFV410_Obj input Bus: SPI_EQ4_OBJ_ELEM_BUS size=20; motionSts output uint8 size=20 =uint8(zeros(20,1)); motionCategory output uint8 size=20 =uint8(zeros(20,1)); motionOrientation output uint8 size=20 =uint8(zeros(20,1))

== matlab function Noa_Nofusion_backup/CR_RSDS_Input/MATLAB Function1 ==
  data: ObjNumber input uint8 size=1; ObjPrio output single size=24; ObjID input uint8 size=24; ObjDx input single size=24; ObjMatrix output single size=24
function [ObjPrio,ObjMatrix] = fcn(ObjNumber,ObjID,ObjDx)
%#codegen
ObjPrio = single(zeros(24,1));

for i=1:ObjNumber
    if ObjID(i)>0
        ObjPrio(i)=single(255) - abs(ObjDx(i));
    else
        ObjPrio(i)=single(0);
    end
end

ObjMatrix=ObjPrio;

t_h=1;
while 1
    t_h = t_h*3+1;
    if t_h>=ObjNumber
        break;
    end
end

%   t_h = 121;
while 1
    t_h = fix(t_h/3);
    for i=(t_h+1):ObjNumber
        j=i;
        t_zw=ObjMatrix(i);
        while (j>t_h)&&(t_zw<ObjMatrix(j-t_h))
            ObjMatrix(j)=ObjMatrix(j-t_h);
            j=j-t_h;
        end
        ObjMatrix(j)=t_zw;
    end
    if t_h==1
        break;
    end
end
end

== matlab function Noa_Nofusion_backup/CR_RSDS_Input/MATLAB Function2 ==
  data: Prio input single size=24; Matrix input single size=24; ID input uint8 size=24; ObjID output uint8 size=11; Dx input single size=24; Dy input single size=24; ObjDx output single size=11; Vx input single size=24; Vy input single size=24; Ax input single size=24; Age input uint8 size=24; MoveSts input uint8 size=24; ObjDy output single size=11; ObjVx output single size=11; ObjVy output single size=11; ObjAx output single size=11; ObjAge output uint8 size=11; ObjMoveSts output uint8 size=11; FusType input uint8 size=24; ObjFusType output uint8 size=11
function [ObjID,ObjDx,ObjDy,ObjVx,ObjVy,ObjAx,ObjAge,ObjMoveSts,ObjFusType] =...
    fcn(Prio,Matrix,ID,Dx,Dy,Vx,Vy,Ax,Age,MoveSts,FusType)
%#codegen
ObjPrioLimit = Matrix(24-11);
ObjID = uint8(zeros(11,1));
ObjDx = single(zeros(11,1));
ObjDy = single(zeros(11,1));
ObjVx = single(zeros(11,1));
ObjVy = single(zeros(11,1));
ObjAx = single(zeros(11,1));
ObjAge = uint8(zeros(11,1));
ObjMoveSts = uint8(zeros(11,1));
ObjFusType = uint8(zeros(11,1));
Num = uint8(0);

for i=1:24
  if ID(i)>0 && Prio(i)>ObjPrioLimit
      Num = Num + uint8(1);
      ObjID(Num) = uint8(i);
      ObjDx(Num) = Dx(i);
      ObjDy(Num) = Dy(i);
      ObjVx(Num) = Vx(i);
      ObjVy(Num) = Vy(i);
      ObjAx(Num) = Ax(i);
      ObjAge(Num) = Age(i);
      ObjMoveSts(Num) = MoveSts(i);
      ObjFusType(Num) = FusType(i);
  end
end

== matlab function Noa_Nofusion_backup/CR_RSDS_Input/RSDS_L_Bus/RSDS_L ==
  data: RadarID input uint8 size=1; ID input uint8 size=6; Dx input single size=6; Dy input single size=6; Vx input single size=6; Vy input single size=6; Ax input single size=6; ObjIDK1 input uint8 size=6; P output uint8 size=6; ObjDx output single size=6; ObjDy output single size=6; ObjVx output single size=6; ObjVy output single size=6; ObjAx output single size=6; ObjMoveSts output uint8 size=6; ObjFusType output uint8 size=6; ObjID output uint8 size=6; ObjAgeK1 input uint8 size=6; ObjAge output uint8 size=6
function [P,ObjDx,ObjDy,ObjVx,ObjVy,ObjAx,ObjMoveSts,ObjFusType,ObjID,ObjAge] =...
    DataT(RadarID,ID,Dx,Dy,Vx,Vy,Ax,ObjIDK1,ObjAgeK1)

if RadarID==uint8(1)
    FusFac = 4;
elseif RadarID==uint8(2)
    FusFac = 8;
elseif RadarID==uint8(3)
    FusFac = 16;
else
    FusFac = 32;
end

ObjID = uint8(zeros(6,1));
ObjDx = single(zeros(6,1));
ObjDy = single(zeros(6,1));
ObjVx = single(zeros(6,1));
ObjVy = single(zeros(6,1));
ObjAx = single(zeros(6,1));
ObjAge = uint8(ones(6,1));
ObjMoveSts = uint8(2*ones(6,1));
ObjFusType = uint8(FusFac*ones(6,1));

T = uint8(zeros(6,1));
P = uint8(zeros(6,1));
Index01 = uint8(zeros(6,1));
Index02 = uint8(zeros(6,1));
M = uint8(0);
N = uint8(0);
w = uint8(0);

for i=uint8(1):uint8(6)
    for j=uint8(1):uint8(6)
        if ID(i)==ObjIDK1(j) && ID(i)>uint8(0)
            T(j) = i;
            P(i) = j;
        end
    end
end

for j=uint8(1):uint8(6)
    if T(j)==uint8(0)
        if ObjIDK1(j)==uint8(0)
            N = N + uint8(1);
            Index01(N) = j;
        else
            M = M + uint8(1);
            Index02(M) = j;
        end
    end
end

for i=uint8(1):uint8(6)
    if P(i)==uint8(0) && ID(i)>uint8(0)
        w = w + uint8(1);
        if w<=N
            P(i) = Index01(w);
        else
            P(i) = Index02(w - N);
        end
    elseif P(i)>uint8(0)
        ObjAge(P(i)) = min(ObjAgeK1(i) + uint8(1),uint8(255));
    end
    if P(i)>uint8(0)
       ObjID(P(i)) = ID(i);
       ObjDx(P(i)) = Dx(i);
       ObjDy(P(i)) = Dy(i);
       ObjVx(P(i)) = Vx(i);
       ObjVy(P(i)) = Vy(i);
       ObjAx(P(i)) = Ax(i);
    end
end
for i=uint8(1):uint8(6)
    if ObjID(i)==uint8(0)
        ObjAge(i) = uint8(0);
        ObjMoveSts(i) = uint8(0);
        ObjFusType(i) = uint8(0);
    end
end
end

== matlab function Noa_Nofusion_backup/CR_RSDS_Input/RSDS_R_Bus/RSDS_R ==
  data: RadarID input uint8 size=1; ID input uint8 size=6; Dx input single size=6; Dy input single size=6; Vx input single size=6; Vy input single size=6; Ax input single size=6; ObjIDK1 input uint8 size=6; P output uint8 size=6; ObjDx output single size=6; ObjDy output single size=6; ObjVx output single size=6; ObjVy output single size=6; ObjAx output single size=6; ObjMoveSts output uint8 size=6; ObjFusType output uint8 size=6; ObjID output uint8 size=6; ObjAgeK1 input uint8 size=6; ObjAge output uint8 size=6
function [P,ObjDx,ObjDy,ObjVx,ObjVy,ObjAx,ObjMoveSts,ObjFusType,ObjID,ObjAge] =...
    DataT(RadarID,ID,Dx,Dy,Vx,Vy,Ax,ObjIDK1,ObjAgeK1)

if RadarID==uint8(1)
    FusFac = 4;
elseif RadarID==uint8(2)
    FusFac = 8;
elseif RadarID==uint8(3)
    FusFac = 16;
else
    FusFac = 32;
end

ObjID = uint8(zeros(6,1));
ObjDx = single(zeros(6,1));
ObjDy = single(zeros(6,1));
ObjVx = single(zeros(6,1));
ObjVy = single(zeros(6,1));
ObjAx = single(zeros(6,1));
ObjAge = uint8(ones(6,1));
ObjMoveSts = uint8(2*ones(6,1));
ObjFusType = uint8(FusFac*ones(6,1));

T = uint8(zeros(6,1));
P = uint8(zeros(6,1));
Index01 = uint8(zeros(6,1));
Index02 = uint8(zeros(6,1));
M = uint8(0);
N = uint8(0);
w = uint8(0);

for i=uint8(1):uint8(6)
    for j=uint8(1):uint8(6)
        if ID(i)==ObjIDK1(j) && ID(i)>uint8(0)
            T(j) = i;
            P(i) = j;
        end
    end
end

for j=uint8(1):uint8(6)
    if T(j)==uint8(0)
        if ObjIDK1(j)==uint8(0)
            N = N + uint8(1);
            Index01(N) = j;
        else
            M = M + uint8(1);
            Index02(M) = j;
        end
    end
end

for i=uint8(1):uint8(6)
    if P(i)==uint8(0) && ID(i)>uint8(0)
        w = w + uint8(1);
        if w<=N
            P(i) = Index01(w);
        else
            P(i) = Index02(w - N);
        end
    elseif P(i)>uint8(0)
        ObjAge(P(i)) = min(ObjAgeK1(i) + uint8(1),uint8(255));
    end
    if P(i)>uint8(0)
       ObjID(P(i)) = ID(i);
       ObjDx(P(i)) = Dx(i);
       ObjDy(P(i)) = Dy(i);
       ObjVx(P(i)) = Vx(i);
       ObjVy(P(i)) = Vy(i);
       ObjAx(P(i)) = Ax(i);
    end
end
for i=uint8(1):uint8(6)
    if ObjID(i)==uint8(0)
        ObjAge(i) = uint8(0);
        ObjMoveSts(i) = uint8(0);
        ObjFusType(i) = uint8(0);
    end
end
end

== matlab function Noa_Nofusion_backup/Subsystem2/ACCOSM/HWA_Task100ms1/OTL1/P0TrajHistCalc01 ==
  data: vRef input; tCycle input single; tSameHandle input single; CutIn input; P0Dx input single; P0Dy input single; P0TrajHistNum output uint8; EgoDDeltaX input single; EgoDDeltaY input single; EgoCosOfPsi input single; EgoSinOfPsi input single; P0TrajHistDxv output single; P0TrajHistDyv output single; P0TrajHistNumK1 input uint8; P0TrajHistDxvK1 input single; P0TrajHistDyvK1 input single
function [P0TrajHistNum,P0TrajHistDxv,P0TrajHistDyv]...
    = fcn(vRef, tCycle,tSameHandle,CutIn, P0Dx,P0Dy,EgoDDeltaX,EgoDDeltaY,EgoCosOfPsi,EgoSinOfPsi,...
    P0TrajHistNumK1,P0TrajHistDxvK1,P0TrajHistDyvK1)
%#codegen
P0TrajHistNum = P0TrajHistNumK1;
P0TrajHistDxv = P0TrajHistDxvK1;
P0TrajHistDyv = P0TrajHistDyvK1;

if tSameHandle==0
    P0TrajHistNum = uint8(0);
    P0TrajHistDxv = single(zeros(24,1));
    P0TrajHistDyv = single(zeros(24,1));
else
    if tSameHandle==tCycle
        if CutIn || (vRef>1)
            P0TrajHistDxv(1) = P0Dx;
            P0TrajHistDyv(1) = P0Dy;
            P0TrajHistNum = uint8(1);
        else
            P0TrajHistDxv(1) = P0Dx;
            P0TrajHistDyv(1) = P0Dy;
            P0TrajHistDxv(2) = P0Dx - single(1);
            P0TrajHistDyv(2) = P0Dy - single(1);
            P0TrajHistDxv(3) = P0Dx - single(2);
            P0TrajHistDyv(3) = P0Dy - single(2);
            P0TrajHistDxv(4) = P0Dx - single(3);
            P0TrajHistDyv(4) = P0Dy - single(3);
            P0TrajHistNum = uint8(4);
        end
    else
        Temp1 = P0TrajHistDxv(1) - EgoDDeltaX - P0Dx;
        Temp2 = P0TrajHistDyv(1) - EgoDDeltaY - P0Dy;
        dDeltaS = Temp1*Temp1 + Temp2*Temp2;
        
        t_d = interpolate(single(8),single(0.5),single(22),single(2.5),single(P0TrajHistNum));
        t_d = t_d*t_d;
        t_AddPosition = (dDeltaS>t_d);
        
        for iBuf=1:P0TrajHistNum
            dX = P0TrajHistDxv(iBuf)-EgoDDeltaX;
            dY = P0TrajHistDyv(iBuf)-EgoDDeltaY;
            P0TrajHistDxv(iBuf) = dX*EgoCosOfPsi + dY*EgoSinOfPsi;
            P0TrajHistDyv(iBuf) = -dX*EgoSinOfPsi + dY*EgoCosOfPsi;
            if (P0TrajHistDxv(iBuf)<-5)||(abs(P0TrajHistDyv(iBuf))>50)
                P0TrajHistNum = max(P0TrajHistNum - uint8(1),uint8(0));
            end
        end
        
        if t_AddPosition==true
            
            P0TrajHistNum = min(P0TrajHistNum + uint8(1),uint8(24));
            for iBuf= P0TrajHistNum:(-1):2
                P0TrajHistDxv(iBuf) = P0TrajHistDxv(iBuf-uint8(1));
                P0TrajHistDyv(iBuf) = P0TrajHistDyv(iBuf-uint8(1));
            end
            P0TrajHistDxv(1) = P0Dx;
            P0TrajHistDyv(1) = P0Dy;
        end
    end
end
end

function out = interpolate(x1,z1,x2,z2,Raw)
if Raw<=x1
    out = z1;
else
    if Raw>=x2
        out = z2;
    else
        out = z1 + (Raw-x1)*(z2-z1)/(x2-x1);
    end
end
end

== matlab function Noa_Nofusion_backup/CSA_Pack/BCMsim ==
  data: SimLeLmp input; CSASim_LampReq output; SimRiLmp input; Model_IDC_L2_LampReq input
function CSASim_LampReq = fcn(SimLeLmp, SimRiLmp, Model_IDC_L2_LampReq)
CSASim_LampReq=Model_IDC_L2_LampReq;
if SimRiLmp
    CSASim_LampReq=uint8(2);
end
if SimLeLmp
    CSASim_LampReq=uint8(1);
end

== matlab function Noa_Nofusion_backup/Subsystem2/ACCOSM/HWA_Task100ms1/OTL1/P0TrajHistCalc1 ==
  data: P0TrajHistNum output uint8; P0TrajHistNum1 input uint8; P0TrajHistDxv1 input single; P0TrajHistDxv output single; P0TrajHistDyv1 input single; P0TrajHistDyv output single; LineValid output boolean; a output single; b output single; c output single; d output single; dxMin output single; dxMax output single
function [P0TrajHistNum,P0TrajHistDxv,P0TrajHistDyv,LineValid,a,b,c,d,dxMin,dxMax] = P0TrajHistMixCalc(...
    P0TrajHistNum1,P0TrajHistDxv1,P0TrajHistDyv1)

P0TrajHistDxv = single(zeros(48,1));
P0TrajHistDyv = single(zeros(48,1));
P0TrajHistNum = uint8(0);

if (P0TrajHistNum1>0)
    P0TrajHistDxv(1:P0TrajHistNum1) = P0TrajHistDxv1(1:P0TrajHistNum1);
    P0TrajHistDyv(1:P0TrajHistNum1) = P0TrajHistDyv1(1:P0TrajHistNum1);
    P0TrajHistNum = P0TrajHistNum1;
end

if P0TrajHistNum>=4
    dxMin = P0TrajHistDxv(P0TrajHistNum);
    dxMax = P0TrajHistDxv(1) + 6;
%     q2 = max(ceil(P0TrajHistNum/2),2);
%     q3 = max(ceil(P0TrajHistNum*3/4),3);
%     q4 = P0TrajHistNum;
%     MaX = [P0TrajHistDxv(1);P0TrajHistDxv(q2);P0TrajHistDxv(q3);P0TrajHistDxv(q4)];
%     MaY = [P0TrajHistDyv(1);P0TrajHistDyv(q2);P0TrajHistDyv(q3);P0TrajHistDyv(q4)];
%     [~,b,c,d] = pl(MaX,MaY);
    P = polyfit(P0TrajHistDxv(1:P0TrajHistNum),P0TrajHistDyv(1:P0TrajHistNum),2);
    b = P(1);
    c = P(2);
    d = P(3);

    a = single(0);
   LineValid = true;
   if dxMin>0.5
      LineValid = false; 
   end
else
   dxMin = single(0); 
   dxMax = single(0); 
   a = single(0);
   b = single(0);
   c = single(0);
   d = single(0);
   LineValid = false;
end

== stateflow chart Noa_Nofusion_backup/CSA_Pack/CSALampCtrlSim/Chart1 ==
  state OFF
    en:
    SwtSts=false;
  state Hold
    en:
    SwtSts=true;
  state LeCloseReady
  (default) -> OFF
  LeCloseReady -> OFF : [SteerWheelAng<P_LmpCloseAngClose...
      | ||OFF]
  Hold -> OFF [order 2] : [OFF]
  OFF -> Hold : [ON]
  Hold -> LeCloseReady [order 1] : [SteerWheelAng>P_LmpCloseAngReady]
  data: SwtSts output; OFF input; ON input; SteerWheelAng input; P_LmpCloseAngClose input; P_LmpCloseAngReady input

== matlab function Noa_Nofusion_backup/Subsystem4/LHLine ==
  data: LH_Count input; LH1A0 input single size=1; LH1A1 input single size=1; LH1A2 input single size=1; LH1A3 input single size=1; LH1RaMin input single size=1; LH1RaMax input single size=1; LH1Conf output uint8 size=1; LH1Avail input uint8 size=1; LH1LineType input uint8 size=1; LH1DLType input uint8 size=1; LH1SideType input uint8 size=1; LH1Wid input single size=1; LH1Crossing input; LH1Confidence input; LH2A0 input single size=1; LH2A1 input single size=1; LH2A2 input single size=1; LH2A3 input single size=1; LH2RaMin input single size=1; LH2RaMax input single size=1; LH2Avail input uint8 size=1; LH2LineType input uint8 size=1; LH2DLType input uint8 size=1; LH2SideType input uint8 size=1; LH2Wid input single size=1; LH1C0 output single size=1; LH1C1 output single size=1; LH1C2 output single size=1; LH1C3 output single size=1; LH1DxMin output single size=1; LH1DxMax output single size=1; LH1Type output uint8 size=1; LH1DLM output uint8 size=1; LH1Width output single size=1; LH1Reliable output; LeftLaneChange output uint8 size=1; LH2Conf output uint8 size=1; LH2C0 output single size=1; LH2C1 output single size=1; LH2C2 output single size=1; LH2C3 output single size=1; LH2DxMin output single size=1; LH2DxMax output single size=1; LH2Type output uint8 size=1; LH2DLM output uint8 size=1; LH2Width output single size=1; LH2Reliable output; RightLaneChange output uint8 size=1; LH2Crossing input; LH2Confidence input
function [LH1Conf,LH1C0,LH1C1,LH1C2,LH1C3,LH1DxMin,LH1DxMax,LH1Type,LH1DLM,LH1Width,LH1Reliable,LeftLaneChange,...
    LH2Conf,LH2C0,LH2C1,LH2C2,LH2C3,LH2DxMin,LH2DxMax,LH2Type,LH2DLM,LH2Width,LH2Reliable,RightLaneChange]...
    = LH(LH_Count,LH1A0,LH1A1,LH1A2,LH1A3,LH1RaMin,LH1RaMax,LH1Avail,LH1LineType,LH1DLType,LH1SideType,LH1Wid,LH1Crossing,LH1Confidence,...
    LH2A0,LH2A1,LH2A2,LH2A3,LH2RaMin,LH2RaMax,LH2Avail,LH2LineType,LH2DLType,LH2SideType,LH2Wid,LH2Crossing,LH2Confidence)

LH1Conf = uint8(0);
LH1C0 = single(0);
LH1C1 = single(0);
LH1C2 = single(0);
LH1C3 = single(0);
LH1DxMin = single(0);
LH1DxMax = single(0);
LH1Type = uint8(0);
LH1DLM = uint8(0);
LH1Width = single(0);
LH1Reliable = single(0);
LeftLaneChange = uint8(0);

LH2Conf = uint8(0);
LH2C0 = single(0);
LH2C1 = single(0);
LH2C2 = single(0);
LH2C3 = single(0);
LH2DxMin = single(0);
LH2DxMax = single(0);
LH2Type = uint8(0);
LH2DLM = uint8(0);
LH2Width = single(0);
LH2Reliable = single(0);
RightLaneChange = uint8(0);


%%
if LH_Count >= 1
    if LH1SideType==1
        LH1Conf = LH1Avail;
        LH1C0 = LH1A0;
        LH1C1 = LH1A1;
        LH1C2 = LH1A2;
        LH1C3 = LH1A3;
        LH1DxMin = LH1RaMin;
        LH1DxMax = LH1RaMax;
        LH1Type = LH1LineType;
        LH1DLM = LH1DLType;
        LH1Width = LH1Wid;
        LH1Reliable = LH1Confidence;
        LeftLaneChange = LH1Crossing;
    elseif LH1SideType==2
        LH2Conf = LH1Avail;
        LH2C0 = LH1A0;
        LH2C1 = LH1A1;
        LH2C2 = LH1A2;
        LH2C3 = LH1A3;
        LH2DxMin = LH1RaMin;
        LH2DxMax = LH1RaMax;
        LH2Type = LH1LineType;
        LH2DLM = LH1DLType;
        LH2Width = LH1Wid;
        LH2Reliable = LH1Confidence;
        RightLaneChange = LH1Crossing;
    end
    if LH_Count >= 2
        if LH2SideType==1
            LH1Conf = LH2Avail;
            LH1C0 = LH2A0;
            LH1C1 = LH2A1;
            LH1C2 = LH2A2;
            LH1C3 = LH2A3;
            LH1DxMin = LH2RaMin;
            LH1DxMax = LH2RaMax;
            LH1Type = LH2LineType;
            LH1DLM = LH2DLType;
            LH1Width = LH2Wid;
            LH1Reliable = LH2Confidence;
            LeftLaneChange = LH2Crossing;
        elseif LH2SideType==2
            LH2Conf = LH2Avail;
            LH2C0 = LH2A0;
            LH2C1 = LH2A1;
            LH2C2 = LH2A2;
            LH2C3 = LH2A3;
            LH2DxMin = LH2RaMin;
            LH2DxMax = LH2RaMax;
            LH2Type = LH2LineType;
            LH2DLM = LH2DLType;
            LH2Width = LH2Wid;
            LH2Reliable = LH2Confidence;
            RightLaneChange = LH2Crossing;
        end
    end
end

== matlab function Noa_Nofusion_backup/Subsystem4/MATLAB Function5 ==
  data: IFV2RearAxis input single size=1; a0 output single size=1; a1 output single size=1; a2 output single size=1; a3 output single size=1; IFV2CenterAxis input single size=1; A0 input single size=1; A1 input single size=1; A2 input single size=1; A3 input single size=1; Range_min input single size=1; Rmin output single size=1; Range_max input single size=1; Rmax output single size=1
function [a0,a1,a2,a3,Rmin,Rmax] = ...
    fcn(IFV2RearAxis,IFV2CenterAxis,A0,A1,A2,A3,Range_min,Range_max)

Rmin = Range_min + IFV2RearAxis;
Rmax = Range_max + IFV2RearAxis;

if Range_max>0
   xi = [10;20;40;80];
   yi = -A3*xi.^3 - A2*xi.^2 - A1*xi - A0 + IFV2CenterAxis;
   xi = xi + IFV2RearAxis;
   [a3,a2,a1,a0] = pl(xi,yi);
else
    a3 = single(0);
    a2 = single(0);
    a1 = single(0);
    a0 = single(0);
end

== matlab function Noa_Nofusion_backup/Subsystem4/MATLAB Function6 ==
  data: IFV2RearAxis input single size=1; a0 output single size=1; a1 output single size=1; a2 output single size=1; a3 output single size=1; IFV2CenterAxis input single size=1; A0 input single size=1; A1 input single size=1; A2 input single size=1; A3 input single size=1; Range_min input single size=1; Rmin output single size=1; Range_max input single size=1; Rmax output single size=1
function [a0,a1,a2,a3,Rmin,Rmax] = ...
    fcn(IFV2RearAxis,IFV2CenterAxis,A0,A1,A2,A3,Range_min,Range_max)

Rmin = Range_min + IFV2RearAxis;
Rmax = Range_max + IFV2RearAxis;

if Range_max>0
   xi = [10;20;40;80];
   yi = -A3*xi.^3 - A2*xi.^2 - A1*xi - A0 + IFV2CenterAxis;
   xi = xi + IFV2RearAxis;
   [a3,a2,a1,a0] = pl(xi,yi);
else
    a3 = single(0);
    a2 = single(0);
    a1 = single(0);
    a0 = single(0);
end

== matlab function Noa_Nofusion_backup/Subsystem4/Simulink Function/MATLAB Function3 ==
  data: IFV2RearAxis input single size=1; a0 output single size=1; a1 output single size=1; a2 output single size=1; a3 output single size=1; IFV2CenterAxis input single size=1; A0 input single size=1; A1 input single size=1; A2 input single size=1; A3 input single size=1; Range_min input single size=1; Rmin output single size=1; Range_max input single size=1; Rmax output single size=1
function [a0,a1,a2,a3,Rmin,Rmax] = ...
    fcn(IFV2RearAxis,IFV2CenterAxis,A0,A1,A2,A3,Range_min,Range_max)

Rmin = Range_min + IFV2RearAxis;
Rmax = Range_max + IFV2RearAxis;

if Range_max>0
   xi = [10;20;40;80];
   yi = -A3*xi.^3 - A2*xi.^2 - A1*xi - A0 + IFV2CenterAxis;
   xi = xi + IFV2RearAxis;
   [a3,a2,a1,a0] = pl(xi,yi);
else
    a3 = single(0);
    a2 = single(0);
    a1 = single(0);
    a0 = single(0);
end

== stateflow chart Noa_Nofusion_backup/CSA_Pack/CSALampCtrlSim/Chart2 ==
  state OFF
    en:
    SwtSts=false;
  state Hold
    en:
    SwtSts=true;
  state LeCloseReady
  (default) -> OFF
  LeCloseReady -> OFF : [abs(SteerWheelAng)>-P_LmpCloseAngClose...
      | ||OFF]
  Hold -> OFF [order 2] : [OFF]
  OFF -> Hold : [ON]
  Hold -> LeCloseReady [order 1] : [SteerWheelAng<-P_LmpCloseAngReady]
  data: SwtSts output; OFF input; ON input; SteerWheelAng input; P_LmpCloseAngClose input; P_LmpCloseAngReady input
